simulink model "plant_cl2"  (Simulink 7.9)
settings: Solver=ode45  StartTime=0.0  StopTime=20  RelTol=1e-3
values from neighbouring files (symbols this model uses):
  d1bar = 0    [script.m]
  d2bar = 0    [script.m]
  Ibar = sign(wbar)*Ifr + b*abs(wbar)*wbar/K + d1bar    [script.m]
  wbar = 300    [script.m]
libraries: cstblocks x1, simulink x1
settings Model: Creator=PhM  LastModifiedBy=PhM
settings OptimizationCC: InitFltsAndDblsToZero=on
settings DebuggingCC: SaveWithParameterizedLinksMsg=none  SignalResolutionControl=TryResolveAllWithWarning  MultiTaskDSMMsg=warning  MultiTaskCondExecSysMsg=none  FcnCallInpInsideContextMsg=Use local settings  StrictBusMsg=None
settings RTWCC: IncludeERTFirstTime=on
settings GRTTargetCC: TargetFcnLib=ansi_tfl_tmw.mat  CombineOutputUpdateFcns=off  GRTInterface=on

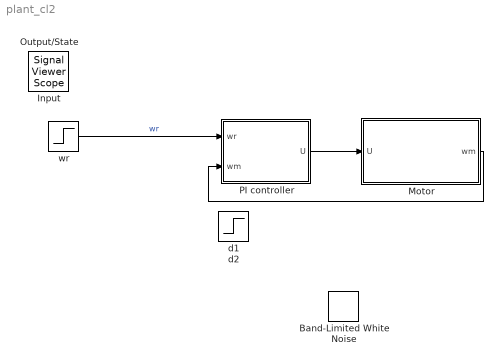
== system plant_cl2 ==
  Motor : Subsystem
  PI controller : Subsystem
  wr : Step  Time=5  Before=wbar  After=wbar+30  SampleTime=0
  Band-Limited White Noise : simulink/Sources/Band-Limited White Noise  IOType=siggen  Cov=1e-2  Ts=1e-2  seed=[23341]
  Input : SignalViewerScope  IOType=viewer  NumInputPorts=3  LegendLocations=|  RefreshTime=0.035000
      | 0.73272     0.91949     0.20122    0.028719
      | 0.72205     0.60805     0.21341    0.028719
      | 0.72205     0.29732     0.21341    0.028719
      settings: ShowLegends=on  TimeRange=20  YMin=4~0~0  YMax=7.5~1~1
  Output/State : SignalViewerScope  IOType=viewer  NumInputPorts=3  RefreshTime=0.035000
      settings: TimeRange=20  YMin=295~295~1.5  YMax=340~335~6
  d1 : Step  IOType=siggen  Time=10  Before=d1bar  After=d1bar+1  SampleTime=0
  d2 : Step  IOType=siggen  Time=15  Before=d2bar  After=d2bar+1  SampleTime=0
  wires:
  wr/1 -> PI controller/1(wr)  "wr"
  PI controller/1(U) -> Motor/1(U)
  Motor/1(wm) -> PI controller/2(wm)

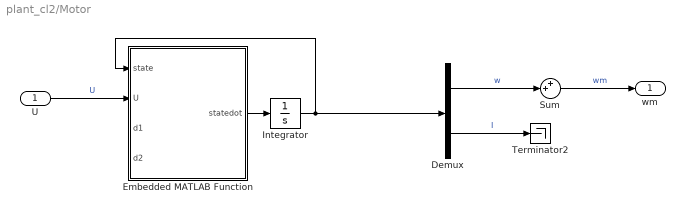
== system plant_cl2/Motor ==
  U : Inport
  Demux : Demux  Outputs=2
  Embedded MATLAB Function : MATLAB Function  TreatAsAtomicUnit=on
  Integrator : Integrator  InitialCondition=[wbar; Ibar]
  Sum : Sum  Inputs=++|
  Terminator2 : Terminator
  wm : Outport
  wires:
  Embedded MATLAB Function/1(statedot) -> Integrator/1
  Integrator/1 -> Embedded MATLAB Function/1(state), Demux/1
  Demux/1 -> Sum/2  "w"
  Demux/2 -> Terminator2/1  "I"
  U/1 -> Embedded MATLAB Function/2(U)  "U"
  Sum/1 -> wm/1  "wm"

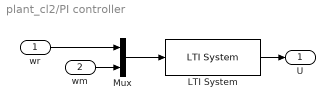
== system plant_cl2/PI controller ==
  wr : Inport
  wm : Inport  Port=2
  LTI System : cstblocks/LTI System  sys=cont  IC=etabar
  Mux : Mux  Inputs=2
  U : Outport
  wires:
  wm/1 -> Mux/2
  LTI System/1 -> U/1
  wr/1 -> Mux/1
  Mux/1 -> LTI System/1

== matlab function Motor/Embedded MATLAB Function ==
  data: state input double; statedot output double; U input double; d1 input double; d2 input double
function statedot = fcn(state,U,d1,d2)
% This block supports an embeddable subset of the MATLAB language.
% See the help menu for details. 

R = 0.56;
L = 4e-3;
Ifr = 0.4;
K = 1.19e-2;
J = 3.45e-5;
b = 2.4e-7;

w = state(1);
I = state(2);

wdot = (K*I  - sign(w)*K*Ifr - b*abs(w)*w - K*d1)/J;
Idot = (-R*I-K*w+U+d2)/L;

statedot = [wdot; Idot];
